simulink model "model_1_Simple_Single_phase_induction_motor"  (R2023b)
settings: Solver=ode23s  StartTime=0.0  StopTime=10.0  MaxStep=1e-4  RelTol=1e-3
undefined symbols (not defined in the file): Capacitor, Run, Start
libraries: spsACVoltageSourceLib x1, spsSinglePhaseAsynchronousMachineLib x1, sps_lib x1
settings Model: Creator=Haier  LastModifiedBy=Haier

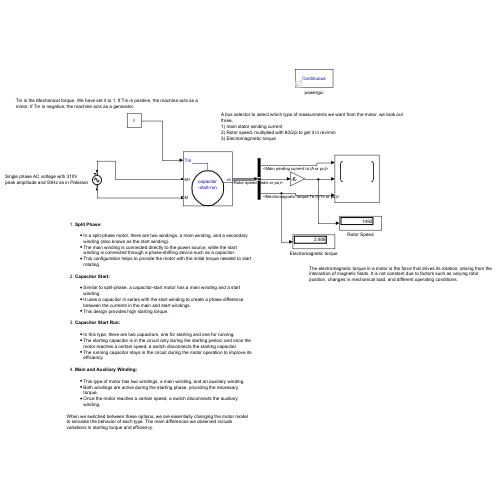
[thumbnail: Simulink's stored preview of the top-level diagram]
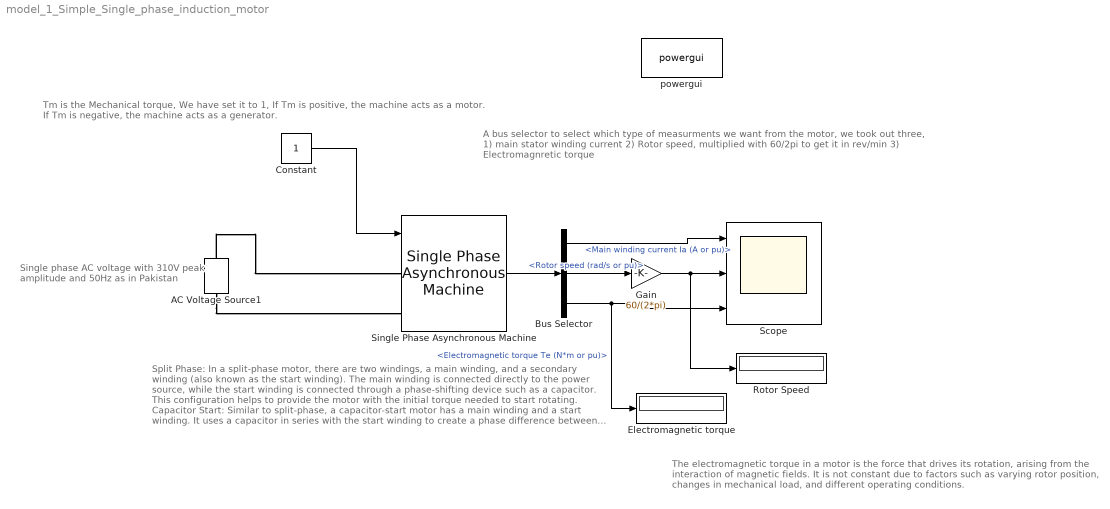
== system model_1_Simple_Single_phase_induction_motor ==
  note: The electromagnetic torque in a motor is the force that drives its rotation, arising from the interaction of magnetic fields. It is not constant due to factors such as varying rotor position, changes in mechanical load, and different operating conditions.
  note: A bus selector to select which type of measurments we want from the motor, we took out three,
      | 1) main stator winding current
      | 2) Rotor speed, multiplied with 60/2pi to get it in rev/min
      | 3) Electromagnretic torque
  note: Split Phase: In a split-phase motor, there are two windings, a main winding, and a secondary winding (also known as the start winding).
      | The main winding is connected directly to the power source, while the start winding is connected through a phase-shifting device such as a capacitor.
      | This configuration helps to provide the motor with the initial torque needed to start rotating.
      |
      | Capacitor Start: Similar to split-phase, a capacitor-start motor has a main winding and a start winding.
      | It uses a capacitor in series with the start winding to create a phase difference between the currents in the main and start windings.
      | This design provides high starting torque.
      |
      | Capacitor Start Run: In this type, there are two capacitors, one for starting and one for running.
      | The starting capacitor is in the circuit only during the starting period, and once the motor reaches a certain speed, a switch disconnects the starting capacitor.
      | The running capacitor stays in the circuit during the motor operation to improve its efficiency.
      |
      | Main and Auxiliary Winding: This type of motor has two windings, a main winding, and an auxiliary winding.
      | Both windings are active during the starting phase, providing the necessary torque.
      | Once the motor reaches a certain speed, a switch disconnects the auxiliary winding.
      |
      | When we switched between these options, we are essentially changing the motor model to simulate the behavior of each type. The main differences we observed include variations in starting torque and efficiency.
  note: Single phase AC voltage with 310V
      | peak amplitude and 50Hz as in Pakistan
  note: Tm is the Mechanical torque, We have set it to 1, If Tm is positive, the machine acts as a motor. If Tm is negative, the machine acts as a generator.
  AC Voltage Source1 : spsACVoltageSourceLib/AC Voltage Source  Amplitude=310  Phase=0  Frequency=50  SampleTime=0  Measurements=None  BusType=swing  Pref=10e3  Qref=0  Qmin=-inf  Qmax=+inf
  Bus Selector : BusSelector  OutputSignals=Stator measurements.Main winding current Ia (A or pu),Mechanical.Rotor speed (rad/s or pu),Mechanical.Electromagnetic torque Te (N*m or pu)
  Constant : Constant
  Electromagnetic torque : Display
  Gain : Gain  Gain=60/(2*pi)
  Rotor Speed : Display
  Scope : Scope  NumInputPorts=3
  Single Phase Asynchronous Machine : spsSinglePhaseAsynchronousMachineLib/Single Phase Asynchronous Machine  MechanicalLoad=Torque Tm  UNITS=SI  MachineType=Capacitor-Start-Run  MeasurementBus=off  NominalParameters="[ .25*746  220  50]"  MainWindingStator="[2.02  7.4e-3]"  MainWindingRotor="[4.12  5.6e-3]"  MutualInductance=0.1772  AuxiliaryWinding="[7.14  8.5e-3]"  Mechanical="[0.0146  0  2 1.18]"  CapacitorStart="[2  254.7e-6]"  CapacitorRun="[18  21.1e-6]"  DisconnectionSpeed=75  InitialSpeed=0  DataType=SI  TsPowergui=0  TsBlock=-1
      settings: LibrarySourceBlock=|
      | sps_lib/Electrical Machines/Single Phase
      | Asynchronous Machine
  powergui : sps_lib/powergui  Priority=1  SimulationMode=Continuous  SampleTime=50e-6  frequency=60  Iterations=50  frequencyindice=50  Pbase=100e6  ErrMax=1e-4  UnitsV=kV  UnitsW=MW  buscounter=0  FunctionMessages=off  echomessages=off  EnableUseOfTLC=off  CurrentSourceSwitches=off  DisableSnubberDevices=off  DisableRonSwitches=off  DisableVfSwitches=off  DisplayEquations=off  AutomaticDiscreteSolvers=off  SolverType=Tustin/Backward Euler (TBE)  Interpol=off  ExternalGateDelay=off  methode=off  Ts=100  x0status=blocks  SPID=on  SwTol=0  HookPort=off  NonlinearTolerance=1e-4  nMaxIteration=100  ContinueOnMaxIteration=off  RestoreLinks=warning  ResistiveCurrentMeasurement=off  Frange=[0:2:500]  Ylog=off  Xlog=on  ShowGrid=off  save=off  variable=ZData  structure=0  ZoomFFT=off  StartTime=0.0  cycles=1  DisplayStyle=1  fundamental=60  FreqAxis=off  MaxFrequency=1000  frequencyindicesteady=1  RmsSteady=1  display=off
  wires:
  Constant/1 -> Single Phase Asynchronous Machine/1
  Single Phase Asynchronous Machine/1 -> Bus Selector/1
  Bus Selector/2 -> Gain/1  "<Rotor speed (rad/s or pu)>"
  Gain/1 -> Rotor Speed/1, Scope/2
  Bus Selector/1 -> Scope/1  "<Main winding current Ia (A or pu)>"
  Bus Selector/3 -> Electromagnetic torque/1, Scope/3  "<Electromagnetic torque Te (N*m or pu)>"
  connections:
  AC Voltage Source1/LConn1 -- Single Phase Asynchronous Machine/LConn2
  AC Voltage Source1/RConn1 -- Single Phase Asynchronous Machine/LConn1
